simulink model "Kalman_measurementData"  (R2019b)
settings: Solver=VariableStepAuto  StartTime=0.0  StopTime=endtime  RelTol=1e-3
values from neighbouring files (symbols this model uses):
  A = [0.01   -0.4940 ; 0.1129 -0.3832]    [Initialization.m]
  B = [0.5919 ; 0.5191]    [Initialization.m]
  C = [1 0]    [Initialization.m]
  ip_excitation = [0 0 0 0 0 0 0 0 0 0 0 0 ... (77 elements, 77x1)]    [measurement_data.mat]
  mn = 0.07    [Initialization.m]
  y_measured = [-0.015158572702 -0.015158572702 -0.0154085014314 -0.0166581450785 -0.0229063633138 -0.0368572658452 -0.0537717888498 -0.0508141342538 -0.0137796068134 0.0232549206271 0.0249718951204 0.025928632948 ... (77 elements, 77x1)]    [measurement_data.mat]
undefined symbols (not defined in the file or in its folder): Continuous, Time
libraries: ctrlSharedLib x1, simulink x1
settings Model: Creator=Devan  LastModifiedBy=Devan

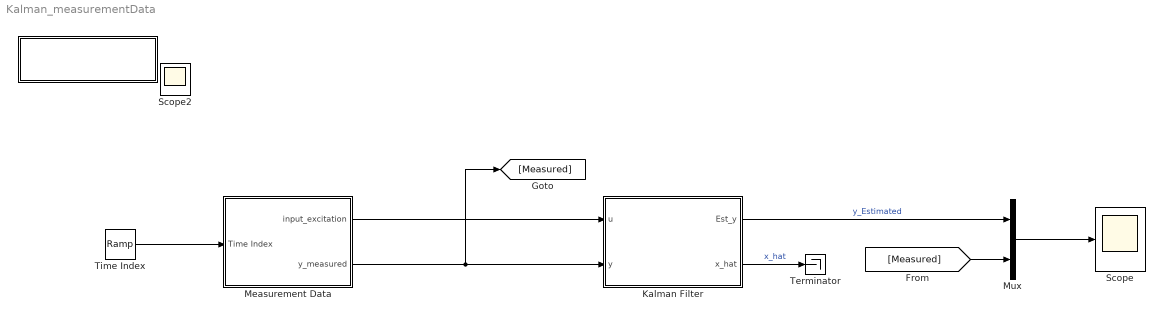
== system Kalman_measurementData ==
  " " : Subsystem  LoadFcn=run('Initialization.m')  InitFcn=run('Initialization.m')
      settings: OpenFcn=run('Initialization.m')
      mask DialogControl Control3 Prompt: Click to Initialize System
      mask Display: disp('Click to Initialize System')
  Kalman Filter : Subsystem
      mask Display: disp('Kalman Filter')
  Measurement Data : Subsystem
      mask Display: disp('MeasurementData')
  Mux : Mux  Inputs=2
  Scope : Scope
  Terminator : Terminator
  Time Index : simulink/Sources/Ramp  slope=1  start=0  InitialOutput=0
  Scope2 : Scope
  wires:
  Mux/1 -> Scope/1
  Kalman Filter/2(x_hat) -> Terminator/1  "x_hat"
  Kalman Filter/1(Est_y) -> Mux/1  "y_Estimated"
  [Measured] -> Mux/2
  Measurement Data/2(y_measured) -> [Measured], Kalman Filter/2(y)
  Time Index/1 -> Measurement Data/1(Time Index)
  Measurement Data/1(input_excitation) -> Kalman Filter/1(u)

== system Kalman_measurementData/  ==

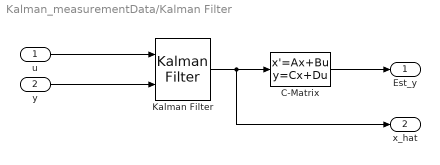
== system Kalman_measurementData/Kalman Filter ==
  u : Inport
  y : Inport  Port=2
  C-Matrix : StateSpace  A=zeros(size(A))  B=zeros(size(A))  C=zeros(size(C))  D=C  InitialCondition=0
  Kalman Filter : ctrlSharedLib/Kalman Filter  TimeDomain=Continuous-Time  UseCurrentEstimator=on  ModelSource=Individual A, B, C, D matrices  ModelSourceVariable=ss(A,B,C,0)  A=A  B=B  C=C  D=0  NumberOfStates=1  NumberOfInputs=1  NumberOfOutputs=1  InitialEstimateSource=Dialog  X0=[0;0]  P0=10  UseK=off  UseGH=off  NumberOfProcessNoiseInputs=1  G=1  TimeInvariantG=on  H=0  TimeInvariantH=on  Q=pn  TimeInvariantQ=on  R=mn  TimeInvariantR=on  N=0  TimeInvariantN=on  AddInputPort=on  AddEnablePort=off  OutputEstimatedY=off  OutputP=off  Ts=-1
      settings: SourceProductBaseCode=CT
  Est_y : Outport
  x_hat : Outport  Port=2
  wires:
  y/1 -> Kalman Filter/2
  Kalman Filter/1 -> x_hat/1, C-Matrix/1
  C-Matrix/1 -> Est_y/1
  u/1 -> Kalman Filter/1

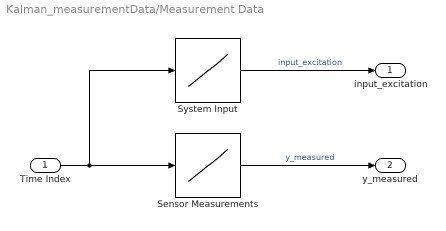
== system Kalman_measurementData/Measurement Data ==
  Time Index : Inport
  Sensor Measurements : Lookup_n-D  NumberOfTableDimensions=1  BreakpointsForDimension1=[1:length(y_measured)]  Table=y_measured([1:length(y_measured)])  InternalRulePriority=Speed  RndMeth=Simplest  InputSameDT=on
  System Input : Lookup_n-D  NumberOfTableDimensions=1  BreakpointsForDimension1=[1:length(y_measured)]  Table=ip_excitation([1:length(y_measured)])  InternalRulePriority=Speed  RndMeth=Simplest  InputSameDT=on
  input_excitation : Outport
  y_measured : Outport  Port=2
  wires:
  Time Index/1 -> System Input/1, Sensor Measurements/1
  Sensor Measurements/1 -> y_measured/1  "y_measured"
  System Input/1 -> input_excitation/1  "input_excitation"
